simulink library "Clock_Lib"  (R2016a)
settings: Solver=ode45  StartTime=0.0  StopTime=10.0  RelTol=1e-3
libraries: simulink_extras x28
settings Model: Creator=Jozko Mrkvicka  LastModifiedBy=Jozko Mrkvicka
settings DataIOCC: LimitDataPoints=on
settings DebuggingCC: AllowSymbolicDim=off

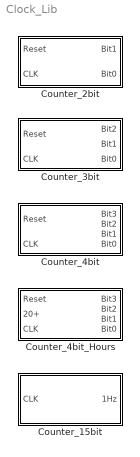
== system Clock_Lib ==
  Counter_15bit : Subsystem
  Counter_2bit : Subsystem
  Counter_3bit : Subsystem
  Counter_4bit : Subsystem
  Counter_4bit_Hours : Subsystem

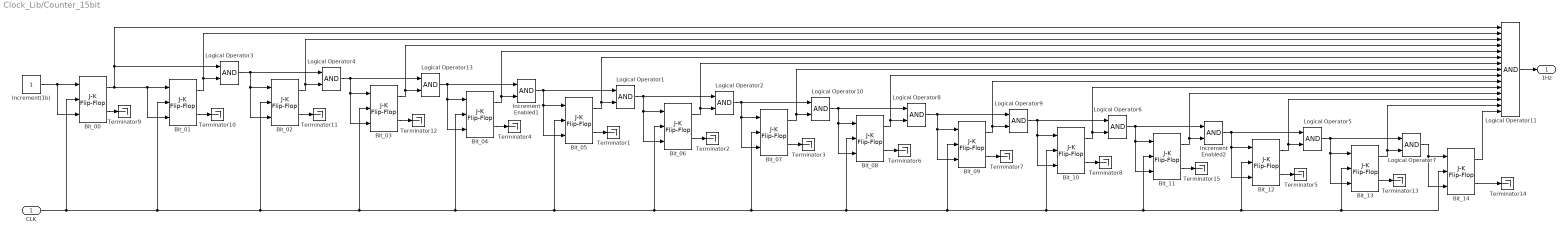
== system Clock_Lib/Counter_15bit ==
  CLK : Inport
  Bit_00 : simulink_extras/Flip Flops/J-K Flip-Flop  initial_condition=0
  Bit_01 : simulink_extras/Flip Flops/J-K Flip-Flop  initial_condition=0
  Bit_02 : simulink_extras/Flip Flops/J-K Flip-Flop  initial_condition=0
  Bit_03 : simulink_extras/Flip Flops/J-K Flip-Flop  initial_condition=0
  Bit_04 : simulink_extras/Flip Flops/J-K Flip-Flop  initial_condition=0
  Bit_05 : simulink_extras/Flip Flops/J-K Flip-Flop  initial_condition=0
  Bit_06 : simulink_extras/Flip Flops/J-K Flip-Flop  initial_condition=0
  Bit_07 : simulink_extras/Flip Flops/J-K Flip-Flop  initial_condition=0
  Bit_08 : simulink_extras/Flip Flops/J-K Flip-Flop  initial_condition=0
  Bit_09 : simulink_extras/Flip Flops/J-K Flip-Flop  initial_condition=0
  Bit_{10..14} (5 alike) : simulink_extras/Flip Flops/J-K Flip-Flop  initial_condition=0
  Increment Enabled1 : Logic  IconShape=distinctive  AllPortsSameDT=off  OutDataTypeStr=boolean
  Increment Enabled2 : Logic  IconShape=distinctive  AllPortsSameDT=off  OutDataTypeStr=boolean
  Increment(1b) : Constant  OutDataTypeStr=boolean
  Logical Operator{1..10,13} (11 alike) : Logic  IconShape=distinctive  AllPortsSameDT=off  OutDataTypeStr=boolean
  Logical Operator11 : Logic  Inputs=15  IconShape=distinctive  AllPortsSameDT=off  OutDataTypeStr=boolean
  Terminator{1..15} (15 alike) : Terminator
  1Hz : Outport
  wires:
  Bit_00/2 -> Terminator9/1
  Increment(1b)/1 -> Bit_00/3, Bit_00/1
  Bit_02/2 -> Terminator11/1
  Bit_03/2 -> Terminator12/1
  Bit_01/2 -> Terminator10/1
  Logical Operator2/1 -> Logical Operator10/1, Bit_07/1, Bit_07/3
  Bit_07/1 -> Logical Operator11/8, Logical Operator10/2
  Bit_06/2 -> Terminator2/1
  Bit_05/2 -> Terminator1/1
  Increment Enabled1/1 -> Bit_05/3, Bit_05/1, Logical Operator1/1
  Bit_07/2 -> Terminator3/1
  Logical Operator13/1 -> Increment Enabled1/1, Bit_04/3, Bit_04/1
  Logical Operator1/1 -> Logical Operator2/1, Bit_06/1, Bit_06/3
  Logical Operator4/1 -> Logical Operator13/1, Bit_03/3, Bit_03/1
  Bit_04/2 -> Terminator4/1
  Logical Operator3/1 -> Logical Operator4/1, Bit_02/3, Bit_02/1
  Bit_09/1 -> Logical Operator11/10, Logical Operator9/2
  Logical Operator10/1 -> Bit_08/1, Bit_08/3, Logical Operator8/1
  Bit_10/1 -> Logical Operator11/11, Logical Operator6/2
  Bit_09/2 -> Terminator7/1
  Bit_10/2 -> Terminator8/1
  Bit_08/2 -> Terminator6/1
  Bit_08/1 -> Logical Operator11/9, Logical Operator8/2
  Bit_13/1 -> Logical Operator11/14, Logical Operator7/2
  Bit_11/1 -> Logical Operator11/12, Increment Enabled2/2
  Bit_12/1 -> Logical Operator11/13, Logical Operator5/2
  Logical Operator7/1 -> Bit_14/1, Bit_14/3
  CLK/1 -> Bit_00/2, Bit_01/2, Bit_02/2, Bit_03/2, Bit_04/2, Bit_05/2, Bit_06/2, Bit_07/2, Bit_08/2, Bit_09/2, Bit_10/2, Bit_11/2, Bit_12/2, Bit_13/2, Bit_14/2
  Bit_14/1 -> Logical Operator11/15
  Bit_13/2 -> Terminator13/1
  Bit_12/2 -> Terminator5/1
  Increment Enabled2/1 -> Bit_12/3, Bit_12/1, Logical Operator5/1
  Bit_14/2 -> Terminator14/1
  Logical Operator6/1 -> Increment Enabled2/1, Bit_11/3, Bit_11/1
  Logical Operator5/1 -> Logical Operator7/1, Bit_13/1, Bit_13/3
  Logical Operator9/1 -> Logical Operator6/1, Bit_10/3, Bit_10/1
  Bit_11/2 -> Terminator15/1
  Logical Operator8/1 -> Logical Operator9/1, Bit_09/3, Bit_09/1
  Bit_06/1 -> Logical Operator11/7, Logical Operator2/2
  Bit_05/1 -> Logical Operator11/6, Logical Operator1/2
  Bit_04/1 -> Logical Operator11/5, Increment Enabled1/2
  Bit_03/1 -> Logical Operator11/4, Logical Operator13/2
  Bit_02/1 -> Logical Operator11/3, Logical Operator4/2
  Bit_01/1 -> Logical Operator11/2, Logical Operator3/2
  Bit_00/1 -> Bit_01/1, Bit_01/3, Logical Operator11/1, Logical Operator3/1
  Logical Operator11/1 -> 1Hz/1

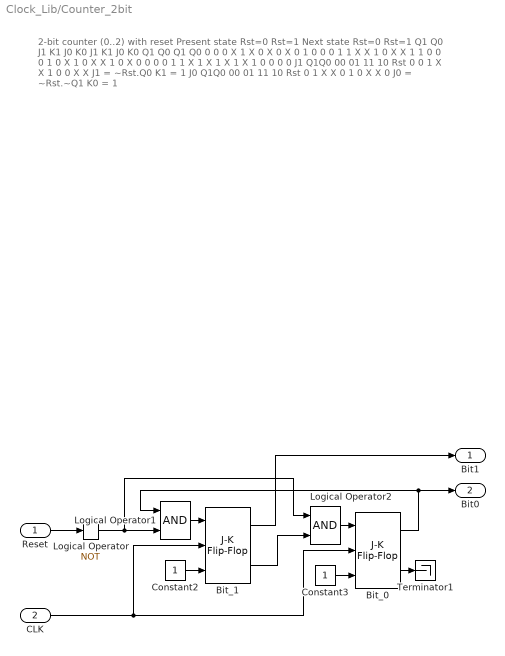
== system Clock_Lib/Counter_2bit ==
  note: 2-bit counter (0..2) with reset
      |
      | Present
      | state
      | Rst=0
      | Rst=1
      | Next state
      |
      | Rst=0
      | Rst=1
      |
      | Q1
      | Q0
      | J1
      | K1
      | J0
      | K0
      | J1
      | K1
      | J0
      | K0
      | Q1
      | Q0
      | Q1
      | Q0
      |
      | 0
      | 0
      | 0
      | X
      | 1
      | X
      | 0
      | X
      | 0
      | X
      | 0
      | 1
      | 0
      | 0
      |
      | 0
      | 1
      | 1
      | X
      | X
      | 1
      | 0
      | X
      | X
      | 1
      | 1
      | 0
      | 0
      | 0
      |
      | 1
      | 0
      | X
      | 1
      | 0
      | X
      | X
      | 1
      | 0
      | X
      | 0
      | 0
      | 0
      | 0
      |
      | 1
      | 1
      | X
      | 1
      | X
      | 1
      | X
      | 1
      | X
      | 1
      | 0
      | 0
      | 0
      | 0
      |
      | J1
      | Q1Q0
      |
      | 00
      | 01
      | 11
      | 10
      |
      | Rst
      | 0
      | 0
      | 1
      | X
      | X
      |
      | 1
      | 0
      | 0
      | X
      | X
      |
      | J1 = ~Rst.Q0
      | K1 = 1
      | J0
      | Q1Q0
      |
      | 00
      | 01
      | 11
      | 10
      |
      | Rst
      | 0
      | 1
      | X
      | X
      | 0
      |
      | 1
      | 0
      | X
      | X
      | 0
      |
      | J0 = ~Rst.~Q1
      | K0 = 1
  Reset : Inport
  CLK : Inport  Port=2
  Bit_0 : simulink_extras/Flip Flops/J-K Flip-Flop  initial_condition=0
  Bit_1 : simulink_extras/Flip Flops/J-K Flip-Flop  initial_condition=0
  Constant2 : Constant  OutDataTypeStr=boolean
  Constant3 : Constant  OutDataTypeStr=boolean
  Logical Operator : Logic  Operator=NOT  IconShape=distinctive  AllPortsSameDT=off  OutDataTypeStr=boolean
  Logical Operator1 : Logic  IconShape=distinctive  AllPortsSameDT=off  OutDataTypeStr=boolean
  Logical Operator2 : Logic  IconShape=distinctive  AllPortsSameDT=off  OutDataTypeStr=boolean
  Terminator1 : Terminator
  Bit1 : Outport
  Bit0 : Outport  Port=2
  wires:
  Constant2/1 -> Bit_1/3
  Constant3/1 -> Bit_0/3
  Bit_0/1 -> Logical Operator1/1, Bit0/1
  Bit_1/2 -> Logical Operator2/2
  CLK/1 -> Bit_0/2, Bit_1/2
  Bit_1/1 -> Bit1/1
  Bit_0/2 -> Terminator1/1
  Logical Operator1/1 -> Bit_1/1
  Reset/1 -> Logical Operator/1
  Logical Operator/1 -> Logical Operator1/2, Logical Operator2/1
  Logical Operator2/1 -> Bit_0/1

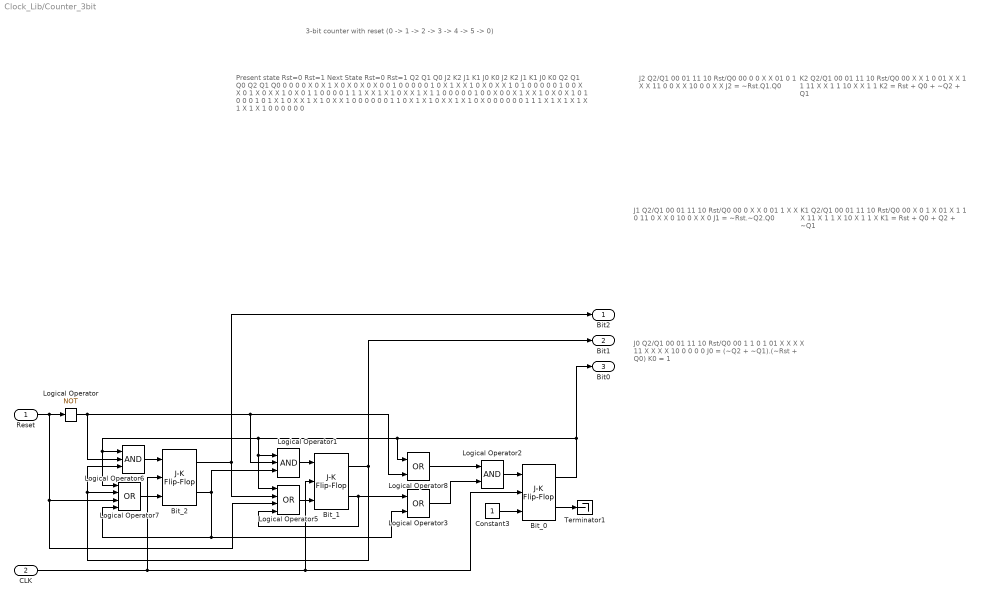
== system Clock_Lib/Counter_3bit ==
  note: J1
      | Q2/Q1
      |
      | 00
      | 01
      | 11
      | 10
      |
      | Rst/Q0
      | 00
      | 0
      | X
      | X
      | 0
      |
      | 01
      | 1
      | X
      | X
      | 0
      |
      | 11
      | 0
      | X
      | X
      | 0
      |
      | 10
      | 0
      | X
      | X
      | 0
      |
      | J1 = ~Rst.~Q2.Q0
  note: J2
      | Q2/Q1
      |
      | 00
      | 01
      | 11
      | 10
      |
      | Rst/Q0
      | 00
      | 0
      | 0
      | X
      | X
      |
      | 01
      | 0
      | 1
      | X
      | X
      |
      | 11
      | 0
      | 0
      | X
      | X
      |
      | 10
      | 0
      | 0
      | X
      | X
      |
      | J2 = ~Rst.Q1.Q0
  note: Present state
      | Rst=0
      | Rst=1
      | Next State
      |
      | Rst=0
      | Rst=1
      |
      | Q2
      | Q1
      | Q0
      | J2
      | K2
      | J1
      | K1
      | J0
      | K0
      | J2
      | K2
      | J1
      | K1
      | J0
      | K0
      | Q2
      | Q1
      | Q0
      | Q2
      | Q1
      | Q0
      |
      | 0
      | 0
      | 0
      | 0
      | X
      | 0
      | X
      | 1
      | X
      | 0
      | X
      | 0
      | X
      | 0
      | X
      | 0
      | 0
      | 1
      | 0
      | 0
      | 0
      |
      | 0
      | 0
      | 1
      | 0
      | X
      | 1
      | X
      | X
      | 1
      | 0
      | X
      | 0
      | X
      | X
      | 1
      | 0
      | 1
      | 0
      | 0
      | 0
      | 0
      |
      | 0
      | 1
      | 0
      | 0
      | X
      | X
      | 0
      | 1
      | X
      | 0
      | X
      | X
      | 1
      | 0
      | X
      | 0
      | 1
      | 1
      | 0
      | 0
      | 0
      |
      | 0
      | 1
      | 1
      | 1
      | X
      | X
      | 1
      | X
      | 1
      | 0
      | X
      | X
      | 1
      | X
      | 1
      | 1
      | 0
      | 0
      | 0
      | 0
      | 0
      |
      | 1
      | 0
      | 0
      | X
      | 0
      | 0
      | X
      | 1
      | X
      | X
      | 1
      | 0
      | X
      | 0
      | X
      | 1
      | 0
      | 1
      | 0
      | 0
      | 0
      |
      | 1
      | 0
      | 1
      | X
      | 1
      | 0
      | X
      | X
      | 1
      | X
      | 1
      | 0
      | X
      | X
      | 1
      | 0
      | 0
      | 0
      | 0
      | 0
      | 0
      |
      | 1
      | 1
      | 0
      | X
      | 1
      | X
      | 1
      | 0
      | X
      | X
      | 1
      | X
      | 1
      | 0
      | X
      | 0
      | 0
      | 0
      | 0
      | 0
      | 0
      |
      | 1
      | 1
      | 1
      | X
      | 1
      | X
      | 1
      | X
      | 1
      | X
      | 1
      | X
      | 1
      | X
      | 1
      | 0
      | 0
      | 0
      | 0
      | 0
      | 0
  note: 3-bit counter with reset
      | (0 -> 1 -> 2 -> 3 -> 4 -> 5 -> 0)
  note: K2
      | Q2/Q1
      |
      | 00
      | 01
      | 11
      | 10
      |
      | Rst/Q0
      | 00
      | X
      | X
      | 1
      | 0
      |
      | 01
      | X
      | X
      | 1
      | 1
      |
      | 11
      | X
      | X
      | 1
      | 1
      |
      | 10
      | X
      | X
      | 1
      | 1
      |
      | K2 = Rst + Q0 + ~Q2 + Q1
  note: K1
      | Q2/Q1
      |
      | 00
      | 01
      | 11
      | 10
      |
      | Rst/Q0
      | 00
      | X
      | 0
      | 1
      | X
      |
      | 01
      | X
      | 1
      | 1
      | X
      |
      | 11
      | X
      | 1
      | 1
      | X
      |
      | 10
      | X
      | 1
      | 1
      | X
      |
      | K1 = Rst + Q0 + Q2 + ~Q1
  note: J0
      | Q2/Q1
      |
      | 00
      | 01
      | 11
      | 10
      |
      | Rst/Q0
      | 00
      | 1
      | 1
      | 0
      | 1
      |
      | 01
      | X
      | X
      | X
      | X
      |
      | 11
      | X
      | X
      | X
      | X
      |
      | 10
      | 0
      | 0
      | 0
      | 0
      |
      | J0 = (~Q2 + ~Q1).(~Rst + Q0)
      | K0 = 1
  Reset : Inport
  CLK : Inport  Port=2
  Bit_0 : simulink_extras/Flip Flops/J-K Flip-Flop  initial_condition=0
  Bit_1 : simulink_extras/Flip Flops/J-K Flip-Flop  initial_condition=0
  Bit_2 : simulink_extras/Flip Flops/J-K Flip-Flop  initial_condition=0
  Constant3 : Constant  OutDataTypeStr=boolean
  Logical Operator : Logic  Operator=NOT  IconShape=distinctive  AllPortsSameDT=off  OutDataTypeStr=boolean
  Logical Operator1 : Logic  Inputs=3  IconShape=distinctive  AllPortsSameDT=off  OutDataTypeStr=boolean
  Logical Operator2 : Logic  IconShape=distinctive  AllPortsSameDT=off  OutDataTypeStr=boolean
  Logical Operator3 : Logic  Operator=OR  IconShape=distinctive  AllPortsSameDT=off  OutDataTypeStr=boolean
  Logical Operator5 : Logic  Operator=OR  Inputs=4  IconShape=distinctive  AllPortsSameDT=off  OutDataTypeStr=boolean
  Logical Operator6 : Logic  Inputs=3  IconShape=distinctive  AllPortsSameDT=off  OutDataTypeStr=boolean
  Logical Operator7 : Logic  Operator=OR  Inputs=4  IconShape=distinctive  AllPortsSameDT=off  OutDataTypeStr=boolean
  Logical Operator8 : Logic  Operator=OR  IconShape=distinctive  AllPortsSameDT=off  OutDataTypeStr=boolean
  Terminator1 : Terminator
  Bit2 : Outport
  Bit1 : Outport  Port=2
  Bit0 : Outport  Port=3
  wires:
  CLK/1 -> Bit_2/2, Bit_1/2, Bit_0/2
  Constant3/1 -> Bit_0/3
  Reset/1 -> Logical Operator/1, Logical Operator5/3, Logical Operator7/3
  Logical Operator/1 -> Logical Operator8/2, Logical Operator1/2, Logical Operator6/2
  Bit_2/1 -> Bit2/1, Logical Operator5/2
  Logical Operator1/1 -> Bit_1/1
  Bit_2/2 -> Logical Operator3/2, Logical Operator7/4, Logical Operator1/3
  Bit_0/1 -> Logical Operator8/1, Logical Operator6/1, Logical Operator7/1, Logical Operator1/1, Logical Operator5/1, Bit0/1
  Logical Operator5/1 -> Bit_1/3
  Bit_1/2 -> Logical Operator3/1, Logical Operator5/4
  Logical Operator6/1 -> Bit_2/1
  Logical Operator7/1 -> Bit_2/3
  Bit_1/1 -> Bit1/1, Logical Operator7/2, Logical Operator6/3
  Logical Operator8/1 -> Logical Operator2/1
  Logical Operator3/1 -> Logical Operator2/2
  Logical Operator2/1 -> Bit_0/1
  Bit_0/2 -> Terminator1/1

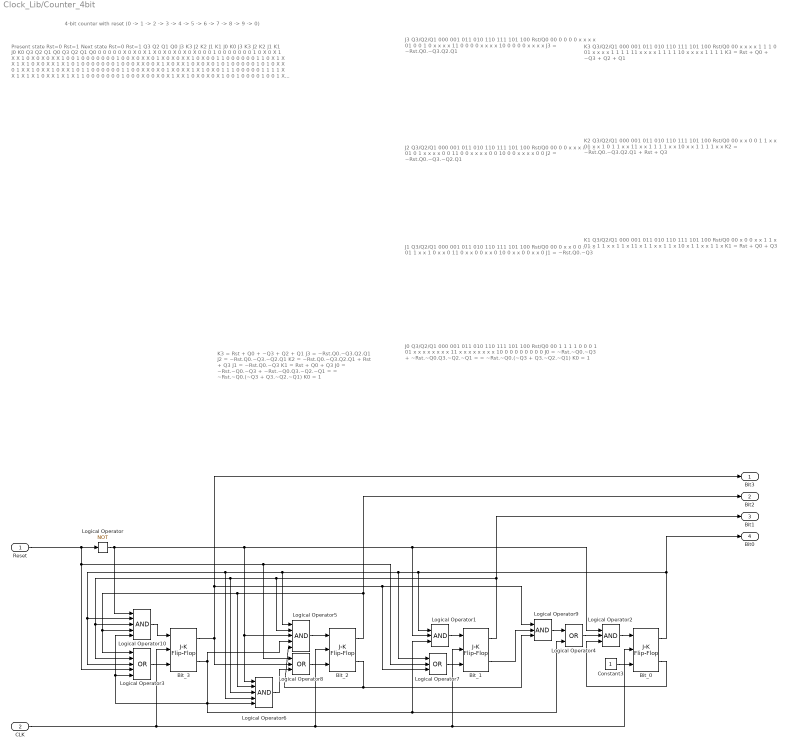
== system Clock_Lib/Counter_4bit ==
  note: K3 = Rst + Q0 + ~Q3 + Q2 + Q1
      | J3 = ~Rst.Q0.~Q3.Q2.Q1
      |
      | J2 = ~Rst.Q0.~Q3.~Q2.Q1
      | K2 = ~Rst.Q0.~Q3.Q2.Q1 + Rst + Q3
      |
      | J1 = ~Rst.Q0.~Q3
      | K1 = Rst + Q0 + Q3
      |
      | J0 = ~Rst.~Q0.~Q3 + ~Rst.~Q0.Q3.~Q2.~Q1 =
      | = ~Rst.~Q0.(~Q3 + Q3.~Q2.~Q1)
      | K0 = 1
  note: Present state
      | Rst=0
      | Rst=1
      | Next state
      |
      | Rst=0
      | Rst=1
      |
      | Q3
      | Q2
      | Q1
      | Q0
      | J3
      | K3
      | J2
      | K2
      | J1
      | K1
      | J0
      | K0
      | J3
      | K3
      | J2
      | K2
      | J1
      | K1
      | J0
      | K0
      | Q3
      | Q2
      | Q1
      | Q0
      | Q3
      | Q2
      | Q1
      | Q0
      |
      | 0
      | 0
      | 0
      | 0
      | 0
      | X
      | 0
      | X
      | 0
      | X
      | 1
      | X
      | 0
      | X
      | 0
      | X
      | 0
      | X
      | 0
      | X
      | 0
      | 0
      | 0
      | 1
      | 0
      | 0
      | 0
      | 0
      |
      | 0
      | 0
      | 0
      | 1
      | 0
      | X
      | 0
      | X
      | 1
      | X
      | X
      | 1
      | 0
      | X
      | 0
      | X
      | 0
      | X
      | X
      | 1
      | 0
      | 0
      | 1
      | 0
      | 0
      | 0
      | 0
      | 0
      |
      | 0
      | 0
      | 1
      | 0
      | 0
      | X
      | 0
      | X
      | X
      | 0
      | 1
      | X
      | 0
      | X
      | 0
      | X
      | X
      | 1
      | 0
      | X
      | 0
      | 0
      | 1
      | 1
      | 0
      | 0
      | 0
      | 0
      |
      | 0
      | 0
      | 1
      | 1
      | 0
      | X
      | 1
      | X
      | X
      | 1
      | X
      | 1
      | 0
      | X
      | 0
      | X
      | X
      | 1
      | X
      | 1
      | 0
      | 1
      | 0
      | 0
      | 0
      | 0
      | 0
      | 0
      |
      | 0
      | 1
      | 0
      | 0
      | 0
      | X
      | X
      | 0
      | 0
      | X
      | 1
      | X
      | 0
      | X
      | X
      | 1
      | 0
      | X
      | 0
      | X
      | 0
      | 1
      | 0
      | 1
      | 0
      | 0
      | 0
      | 0
      |
      | 0
      | 1
      | 0
      | 1
      | 0
      | X
      | X
      | 0
      | 1
      | X
      | X
      | 1
      | 0
      | X
      | X
      | 1
      | 0
      | X
      | X
      | 1
      | 0
      | 1
      | 1
      | 0
      | 0
      | 0
      | 0
      | 0
      |
      | 0
      | 1
      | 1
      | 0
      | 0
      | X
      | X
      | 0
      | X
      | 0
      | 1
      | X
      | 0
      | X
      | X
      | 1
      | X
      | 1
      | 0
      | X
      | 0
      | 1
      | 1
      | 1
      | 0
      | 0
      | 0
      | 0
      |
      | 0
      | 1
      | 1
      | 1
      | 1
      | X
      | X
      | 1
      | X
      | 1
      | X
      | 1
      | 0
      | X
      | X
      | 1
      | X
      | 1
      | X
      | 1
      | 1
      | 0
      | 0
      | 0
      | 0
      | 0
      | 0
      | 0
      |
      | 1
      | 0
      | 0
      | 0
      | X
      | 0
      | 0
      | X
      | 0
      | X
      | 1
      | X
      | X
      | 1
      | 0
      | X
      | 0
      | X
      | 0
      | X
      | 1
      | 0
      | 0
      | 1
      | 0
      | 0
      | 0
      | 0
      |
      | 1
      | 0
      | 0
      | 1
      | X
      | 1
      | 0
      | X
      | 0
      | X
      | X
      | 1
      | X
      | 1
      | 0
      | X
      | 0
      | X
      | X
      | 1
      | 0
      | 0
      | 0
      | 0
      | 0
      | 0
      | 0
      | 0
      |
      | 1
      | 0
      | 1
      | 0
      | X
      | 1
      | 0
      | X
      | X
      | 1
      | 0
      | X
      | X
      | 1
      | 0
      | X
      | X
      | 1
      | 0
      | X
      | 0
      | 0
      | 0
      | 0
      | 0
      | 0
      | 0
      | 0
      |
      | 1
      | 0
      | 1
      | 1
      | X
      | 1
      | 0
      | X
      | X
      | 1
      | X
      | 1
      | X
      | 1
      | 0
      | X
      | X
      | 1
      | X
      | 1
      | 0
      | 0
      | 0
      | 0
      | 0
      | 0
      | 0
      | 0
      |
      | 1
      | 1
      | 0
      | 0
      | X
      | 1
      | X
      | 1
      | 0
      | X
      | 0
      | X
      | X
      | 1
      | X
      | 1
      | 0
      | X
      | 0
      | X
      | 0
      | 0
      | 0
      | 0
      | 0
      | 0
      | 0
      | 0
      |
      | 1
      | 1
      | 0
      | 1
      | X
      | 1
      | X
      | 1
      | 0
      | X
      | X
      | 1
      | X
      | 1
      | X
      | 1
      | 0
      | X
      | X
      | 1
      | 0
      | 0
      | 0
      | 0
      | 0
      | 0
      | 0
      | 0
      |
      | 1
      | 1
      | 1
      | 0
      | X
      | 1
      | X
      | 1
      | X
      | 1
      | 0
      | X
      | X
      | 1
      | X
      | 1
      | X
      | 1
      | 0
      | X
      | 0
      | 0
      | 0
      | 0
      | 0
      | 0
      | 0
      | 0
      |
      | 1
      | 1
      | 1
      | 1
      | X
      | 1
      | X
      | 1
      | X
      | 1
      | X
      | 1
      | X
      | 1
      | X
      | 1
      | X
      | 1
      | X
      | 1
      | 0
      | 0
      | 0
      | 0
      | 0
      | 0
      | 0
      | 0
  note: 4-bit counter with reset
      | (0 -> 1 -> 2 -> 3 -> 4 -> 5 -> 6 -> 7 -> 8 -> 9 -> 0)
  note: K3
      | Q3/Q2/Q1
      |
      | 000
      | 001
      | 011
      | 010
      | 110
      | 111
      | 101
      | 100
      |
      | Rst/Q0
      | 00
      | x
      | x
      | x
      | x
      | 1
      | 1
      | 1
      | 0
      |
      | 01
      | x
      | x
      | x
      | x
      | 1
      | 1
      | 1
      | 1
      |
      | 11
      | x
      | x
      | x
      | x
      | 1
      | 1
      | 1
      | 1
      |
      | 10
      | x
      | x
      | x
      | x
      | 1
      | 1
      | 1
      | 1
      |
      | K3 = Rst + Q0 + ~Q3 + Q2 + Q1
  note: J2
      | Q3/Q2/Q1
      |
      | 000
      | 001
      | 011
      | 010
      | 110
      | 111
      | 101
      | 100
      |
      | Rst/Q0
      | 00
      | 0
      | 0
      | x
      | x
      | x
      | x
      | 0
      | 0
      |
      | 01
      | 0
      | 1
      | x
      | x
      | x
      | x
      | 0
      | 0
      |
      | 11
      | 0
      | 0
      | x
      | x
      | x
      | x
      | 0
      | 0
      |
      | 10
      | 0
      | 0
      | x
      | x
      | x
      | x
      | 0
      | 0
      |
      | J2 = ~Rst.Q0.~Q3.~Q2.Q1
  note: K2
      | Q3/Q2/Q1
      |
      | 000
      | 001
      | 011
      | 010
      | 110
      | 111
      | 101
      | 100
      |
      | Rst/Q0
      | 00
      | x
      | x
      | 0
      | 0
      | 1
      | 1
      | x
      | x
      |
      | 01
      | x
      | x
      | 1
      | 0
      | 1
      | 1
      | x
      | x
      |
      | 11
      | x
      | x
      | 1
      | 1
      | 1
      | 1
      | x
      | x
      |
      | 10
      | x
      | x
      | 1
      | 1
      | 1
      | 1
      | x
      | x
      |
      | K2 = ~Rst.Q0.~Q3.Q2.Q1 + Rst + Q3
  note: J1
      | Q3/Q2/Q1
      |
      | 000
      | 001
      | 011
      | 010
      | 110
      | 111
      | 101
      | 100
      |
      | Rst/Q0
      | 00
      | 0
      | x
      | x
      | 0
      | 0
      | x
      | x
      | 0
      |
      | 01
      | 1
      | x
      | x
      | 1
      | 0
      | x
      | x
      | 0
      |
      | 11
      | 0
      | x
      | x
      | 0
      | 0
      | x
      | x
      | 0
      |
      | 10
      | 0
      | x
      | x
      | 0
      | 0
      | x
      | x
      | 0
      |
      | J1 = ~Rst.Q0.~Q3
  note: K1
      | Q3/Q2/Q1
      |
      | 000
      | 001
      | 011
      | 010
      | 110
      | 111
      | 101
      | 100
      |
      | Rst/Q0
      | 00
      | x
      | 0
      | 0
      | x
      | x
      | 1
      | 1
      | x
      |
      | 01
      | x
      | 1
      | 1
      | x
      | x
      | 1
      | 1
      | x
      |
      | 11
      | x
      | 1
      | 1
      | x
      | x
      | 1
      | 1
      | x
      |
      | 10
      | x
      | 1
      | 1
      | x
      | x
      | 1
      | 1
      | x
      |
      | K1 = Rst + Q0 + Q3
  note: J0
      | Q3/Q2/Q1
      |
      | 000
      | 001
      | 011
      | 010
      | 110
      | 111
      | 101
      | 100
      |
      | Rst/Q0
      | 00
      | 1
      | 1
      | 1
      | 1
      | 0
      | 0
      | 0
      | 1
      |
      | 01
      | x
      | x
      | x
      | x
      | x
      | x
      | x
      | x
      |
      | 11
      | x
      | x
      | x
      | x
      | x
      | x
      | x
      | x
      |
      | 10
      | 0
      | 0
      | 0
      | 0
      | 0
      | 0
      | 0
      | 0
      |
      | J0 = ~Rst.~Q0.~Q3 + ~Rst.~Q0.Q3.~Q2.~Q1 =
      | = ~Rst.~Q0.(~Q3 + Q3.~Q2.~Q1)
      | K0 = 1
  note: J3
      | Q3/Q2/Q1
      |
      | 000
      | 001
      | 011
      | 010
      | 110
      | 111
      | 101
      | 100
      |
      | Rst/Q0
      | 00
      | 0
      | 0
      | 0
      | 0
      | x
      | x
      | x
      | x
      |
      | 01
      | 0
      | 0
      | 1
      | 0
      | x
      | x
      | x
      | x
      |
      | 11
      | 0
      | 0
      | 0
      | 0
      | x
      | x
      | x
      | x
      |
      | 10
      | 0
      | 0
      | 0
      | 0
      | x
      | x
      | x
      | x
      |
      | J3 = ~Rst.Q0.~Q3.Q2.Q1
  Reset : Inport
  CLK : Inport  Port=2
  Bit_{0..3} (4 alike) : simulink_extras/Flip Flops/J-K Flip-Flop  initial_condition=0
  Constant3 : Constant  OutDataTypeStr=boolean
  Logical Operator : Logic  Operator=NOT  IconShape=distinctive  AllPortsSameDT=off  OutDataTypeStr=boolean
  Logical Operator1 : Logic  Inputs=3  IconShape=distinctive  AllPortsSameDT=off  OutDataTypeStr=boolean
  Logical Operator10 : Logic  Inputs=5  IconShape=distinctive  AllPortsSameDT=off  OutDataTypeStr=boolean
  Logical Operator2 : Logic  Inputs=3  IconShape=distinctive  AllPortsSameDT=off  OutDataTypeStr=boolean
  Logical Operator3 : Logic  Operator=OR  Inputs=5  IconShape=distinctive  AllPortsSameDT=off  OutDataTypeStr=boolean
  Logical Operator4 : Logic  Operator=OR  IconShape=distinctive  AllPortsSameDT=off  OutDataTypeStr=boolean
  Logical Operator5 : Logic  Inputs=5  IconShape=distinctive  AllPortsSameDT=off  OutDataTypeStr=boolean
  Logical Operator6 : Logic  Inputs=5  IconShape=distinctive  AllPortsSameDT=off  OutDataTypeStr=boolean
  Logical Operator7 : Logic  Operator=OR  Inputs=3  IconShape=distinctive  AllPortsSameDT=off  OutDataTypeStr=boolean
  Logical Operator8 : Logic  Operator=OR  Inputs=3  IconShape=distinctive  AllPortsSameDT=off  OutDataTypeStr=boolean
  Logical Operator9 : Logic  Inputs=3  IconShape=distinctive  AllPortsSameDT=off  OutDataTypeStr=boolean
  Bit3 : Outport
  Bit2 : Outport  Port=2
  Bit1 : Outport  Port=3
  Bit0 : Outport  Port=4
  wires:
  CLK/1 -> Bit_3/2, Bit_2/2, Bit_1/2, Bit_0/2
  Constant3/1 -> Bit_0/3
  Logical Operator10/1 -> Bit_3/1
  Logical Operator3/1 -> Bit_3/3
  Bit_3/2 -> Logical Operator5/4, Logical Operator1/3, Logical Operator4/2, Logical Operator6/5, Logical Operator3/5, Logical Operator10/5
  Bit_2/1 -> Bit2/1, Logical Operator6/2, Logical Operator3/1, Logical Operator10/4
  Bit_0/1 -> Bit0/1, Logical Operator1/1, Logical Operator7/1, Logical Operator5/1, Logical Operator6/4, Logical Operator10/2, Logical Operator3/3
  Logical Operator/1 -> Logical Operator10/1, Logical Operator2/1, Logical Operator1/2, Logical Operator5/3, Logical Operator6/1
  Logical Operator5/1 -> Bit_2/1
  Bit_2/2 -> Logical Operator5/5, Logical Operator9/3
  Logical Operator8/1 -> Bit_2/3
  Bit_3/1 -> Bit3/1, Logical Operator7/3, Logical Operator9/1, Logical Operator8/2
  Logical Operator6/1 -> Logical Operator8/3
  Bit_1/1 -> Bit1/1, Logical Operator5/2, Logical Operator10/3, Logical Operator3/2, Logical Operator6/3
  Logical Operator1/1 -> Bit_1/1
  Logical Operator7/1 -> Bit_1/3
  Reset/1 -> Logical Operator/1, Logical Operator7/2, Logical Operator8/1, Logical Operator3/4
  Logical Operator4/1 -> Logical Operator2/2
  Logical Operator2/1 -> Bit_0/1
  Bit_0/2 -> Logical Operator2/3
  Logical Operator9/1 -> Logical Operator4/1
  Bit_1/2 -> Logical Operator9/2

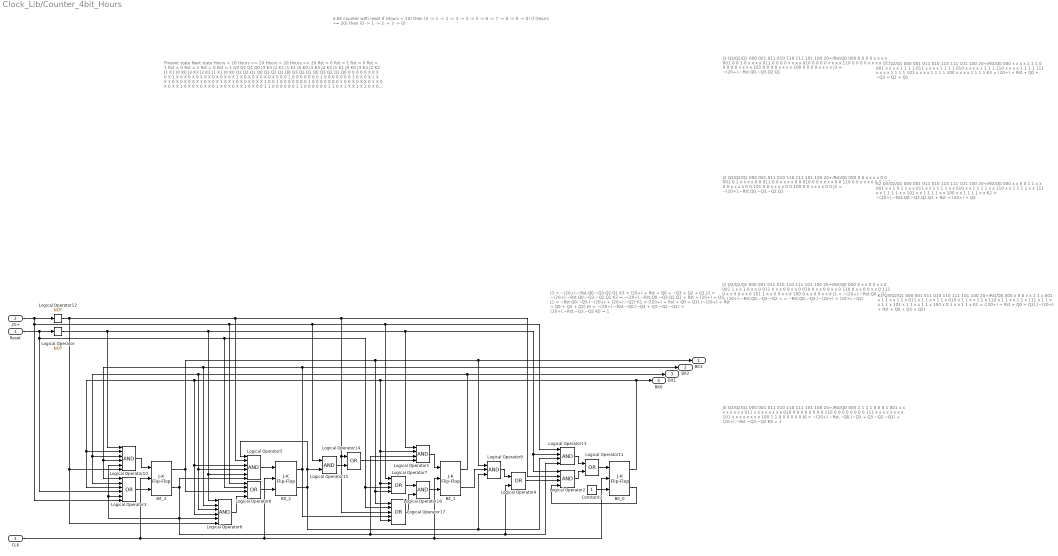
== system Clock_Lib/Counter_4bit_Hours ==
  note: J3 = ~(20+).~Rst.Q0.~Q3.Q2.Q1
      | K3 = (20+) + Rst + Q0 + ~Q3 + Q2 + Q1
      |
      | J2 = ~(20+).~Rst.Q0.~Q3.~Q2.Q1
      | K2 = ~(20+).~Rst.Q0.~Q3.Q2.Q1 + Rst + (20+) + Q3
      |
      | J1 = ~Rst.Q0.~Q3.(~(20+) + (20+).~Q2)
      | K1 = ((20+) + Rst + Q0 + Q3).(~(20+) + Rst + Q0 + Q3 + Q2)
      |
      | J0 = ~(20+).~Rst.~Q0.(~Q3 + Q3.~Q2.~Q1) + (20+).~Rst.~Q3.~Q2
      | K0 = 1
  note: Present state
      |
      | Next state
      |
      | Hours < 20
      | Hours >= 20
      | Hours < 20
      | Hours >= 20
      |
      | Rst = 0
      | Rst = 1
      | Rst = 0
      | Rst = 1
      | Rst = 0
      | Rst = 1
      | Rst = 0
      | Rst = 1
      |
      | Q3
      | Q2
      | Q1
      | Q0
      | J3
      | K3
      | J2
      | K2
      | J1
      | K1
      | J0
      | K0
      | J3
      | K3
      | J2
      | K2
      | J1
      | K1
      | J0
      | K0
      | J3
      | K3
      | J2
      | K2
      | J1
      | K1
      | J0
      | K0
      | J3
      | K3
      | J2
      | K2
      | J1
      | K1
      | J0
      | K0
      | Q3
      | Q2
      | Q1
      | Q0
      | Q3
      | Q2
      | Q1
      | Q0
      | Q3
      | Q2
      | Q1
      | Q0
      | Q3
      | Q2
      | Q1
      | Q0
      |
      | 0
      | 0
      | 0
      | 0
      | 0
      | X
      | 0
      | X
      | 0
      | X
      | 1
      | X
      | 0
      | X
      | 0
      | X
      | 0
      | X
      | 0
      | X
      | 0
      | X
      | 0
      | X
      | 0
      | X
      | 1
      | X
      | 0
      | X
      | 0
      | X
      | 0
      | X
      | 0
      | X
      | 0
      | 0
      | 0
      | 1
      | 0
      | 0
      | 0
      | 0
      | 0
      | 0
      | 0
      | 1
      | 0
      | 0
      | 0
      | 0
      |
      | 0
      | 0
      | 0
      | 1
      | 0
      | X
      | 0
      | X
      | 1
      | X
      | X
      | 1
      | 0
      | X
      | 0
      | X
      | 0
      | X
      | X
      | 1
      | 0
      | X
      | 0
      | X
      | 1
      | X
      | X
      | 1
      | 0
      | X
      | 0
      | X
      | 0
      | X
      | X
      | 1
      | 0
      | 0
      | 1
      | 0
      | 0
      | 0
      | 0
      | 0
      | 0
      | 0
      | 1
      | 0
      | 0
      | 0
      | 0
      | 0
      |
      | 0
      | 0
      | 1
      | 0
      | 0
      | X
      | 0
      | X
      | X
      | 0
      | 1
      | X
      | 0
      | X
      | 0
      | X
      | X
      | 1
      | 0
      | X
      | 0
      | X
      | 0
      | X
      | X
      | 0
      | 1
      | X
      | 0
      | X
      | 0
      | X
      | X
      | 1
      | 0
      | X
      | 0
      | 0
      | 1
      | 1
      | 0
      | 0
      | 0
      | 0
      | 0
      | 0
      | 1
      | 1
      | 0
      | 0
      | 0
      | 0
      |
      | 0
      | 0
      | 1
      | 1
      | 0
      | X
      | 1
      | X
      | X
      | 1
      | X
      | 1
      | 0
      | X
      | 0
      | X
      | X
      | 1
      | X
      | 1
      | 0
      | X
      | 0
      | X
      | X
      | 1
      | X
      | 1
      | 0
      | X
      | 0
      | X
      | X
      | 1
      | X
      | 1
      | 0
      | 1
      | 0
      | 0
      | 0
      | 0
      | 0
      | 0
      | 0
      | 0
      | 0
      | 0
      | 0
      | 0
      | 0
      | 0
      |
      | 0
      | 1
      | 0
      | 0
      | 0
      | X
      | X
      | 0
      | 0
      | X
      | 1
      | X
      | 0
      | X
      | X
      | 1
      | 0
      | X
      | 0
      | X
      | 0
      | X
      | X
      | 1
      | 0
      | X
      | 0
      | X
      | 0
      | X
      | X
      | 1
      | 0
      | X
      | 0
      | X
      | 0
      | 1
      | 0
      | 1
      | 0
      | 0
      | 0
      | 0
      | 0
      | 0
      | 0
      | 0
      | 0
      | 0
      | 0
      | 0
      |
      | 0
      | 1
      | 0
      | 1
      | 0
      | X
      | X
      | 0
      | 1
      | X
      | X
      | 1
      | 0
      | X
      | X
      | 1
      | 0
      | X
      | X
      | 1
      | 0
      | X
      | X
      | 1
      | 0
      | X
      | X
      | 1
      | 0
      | X
      | X
      | 1
      | 0
      | X
      | X
      | 1
      | 0
      | 1
      | 1
      | 0
      | 0
      | 0
      | 0
      | 0
      | 0
      | 0
      | 0
      | 0
      | 0
      | 0
      | 0
      | 0
      |
      | 0
      | 1
      | 1
      | 0
      | 0
      | X
      | X
      | 0
      | X
      | 0
      | 1
      | X
      | 0
      | X
      | X
      | 1
      | X
      | 1
      | 0
      | X
      | 0
      | X
      | X
      | 1
      | X
      | 1
      | 0
      | X
      | 0
      | X
      | X
      | 1
      | X
      | 1
      | 0
      | X
      | 0
      | 1
      | 1
      | 1
      | 0
      | 0
      | 0
      | 0
      | 0
      | 0
      | 0
      | 0
      | 0
      | 0
      | 0
      | 0
      |
      | 0
      | 1
      | 1
      | 1
      | 1
      | X
      | X
      | 1
      | X
      | 1
      | X
      | 1
      | 0
      | X
      | X
      | 1
      | X
      | 1
      | X
      | 1
      | 0
      | X
      | X
      | 1
      | X
      | 1
      | X
      | 1
      | 0
      | X
      | X
      | 1
      | X
      | 1
      | X
      | 1
      | 1
      | 0
      | 0
      | 0
      | 0
      | 0
      | 0
      | 0
      | 0
      | 0
      | 0
      | 0
      | 0
      | 0
      | 0
      | 0
      |
      | 1
      | 0
      | 0
      | 0
      | X
      | 0
      | 0
      | X
      | 0
      | X
      | 1
      | X
      | X
      | 1
      | 0
      | X
      | 0
      | X
      | 0
      | X
      | X
      | 1
      | 0
      | X
      | 0
      | X
      | 0
      | X
      | X
      | 1
      | 0
      | X
      | 0
      | X
      | 0
      | X
      | 1
      | 0
      | 0
      | 1
      | 0
      | 0
      | 0
      | 0
      | 0
      | 0
      | 0
      | 0
      | 0
      | 0
      | 0
      | 0
      |
      | 1
      | 0
      | 0
      | 1
      | X
      | 1
      | 0
      | X
      | 0
      | X
      | X
      | 1
      | X
      | 1
      | 0
      | X
      | 0
      | X
      | X
      | 1
      | X
      | 1
      | 0
      | X
      | 0
      | X
      | X
      | 1
      | X
      | 1
      | 0
      | X
      | 0
      | X
      | X
      | 1
      | 0
      | 0
      | 0
      | 0
      | 0
      | 0
      | 0
      | 0
      | 0
      | 0
      | 0
      | 0
      | 0
      | 0
      | 0
      | 0
      |
      | 1
      | 0
      | 1
      | 0
      | X
      | 1
      | 0
      | X
      | X
      | 1
      | 0
      | X
      | X
      | 1
      | 0
      | X
      | X
      | 1
      | 0
      | X
      | X
      | 1
      | 0
      | X
      | X
      | 1
      | 0
      | X
      | X
      | 1
      | 0
      | X
      | X
      | 1
      | 0
      | X
      | 0
      | 0
      | 0
      | 0
      | 0
      | 0
      | 0
      | 0
      | 0
      | 0
      | 0
      | 0
      | 0
      | 0
      | 0
      | 0
      |
      | 1
      | 0
      | 1
      | 1
      | X
      | 1
      | 0
      | X
      | X
      | 1
      | X
      | 1
      | X
      | 1
      | 0
      | X
      | X
      | 1
      | X
      | 1
      | X
      | 1
      | 0
      | X
      | X
      | 1
      | X
      | 1
      | X
      | 1
      | 0
      | X
      | X
      | 1
      | X
      | 1
      | 0
      | 0
      | 0
      | 0
      | 0
      | 0
      | 0
      | 0
      | 0
      | 0
      | 0
      | 0
      | 0
      | 0
      | 0
      | 0
      |
      | 1
      | 1
      | 0
      | 0
      | X
      | 1
      | X
      | 1
      | 0
      | X
      | 0
      | X
      | X
      | 1
      | X
      | 1
      | 0
      | X
      | 0
      | X
      | X
      | 1
      | X
      | 1
      | 0
      | X
      | 0
      | X
      | X
      | 1
      | X
      | 1
      | 0
      | X
      | 0
      | X
      | 0
      | 0
      | 0
      | 0
      | 0
      | 0
      | 0
      | 0
      | 0
      | 0
      | 0
      | 0
      | 0
      | 0
      | 0
      | 0
      |
      | 1
      | 1
      | 0
      | 1
      | X
      | 1
      | X
      | 1
      | 0
      | X
      | X
      | 1
      | X
      | 1
      | X
      | 1
      | 0
      | X
      | X
      | 1
      | X
      | 1
      | X
      | 1
      | 0
      | X
      | X
      | 1
      | X
      | 1
      | X
      | 1
      | 0
      | X
      | X
      | 1
      | 0
      | 0
      | 0
      | 0
      | 0
      | 0
      | 0
      | 0
      | 0
      | 0
      | 0
      | 0
      | 0
      | 0
      | 0
      | 0
      |
      | 1
      | 1
      | 1
      | 0
      | X
      | 1
      | X
      | 1
      | X
      | 1
      | 0
      | X
      | X
      | 1
      | X
      | 1
      | X
      | 1
      | 0
      | X
      | X
      | 1
      | X
      | 1
      | X
      | 1
      | 0
      | X
      | X
      | 1
      | X
      | 1
      | X
      | 1
      | 0
      | X
      | 0
      | 0
      | 0
      | 0
      | 0
      | 0
      | 0
      | 0
      | 0
      | 0
      | 0
      | 0
      | 0
      | 0
      | 0
      | 0
      |
      | 1
      | 1
      | 1
      | 1
      | X
      | 1
      | X
      | 1
      | X
      | 1
      | X
      | 1
      | X
      | 1
      | X
      | 1
      | X
      | 1
      | X
      | 1
      | X
      | 1
      | X
      | 1
      | X
      | 1
      | X
      | 1
      | X
      | 1
      | X
      | 1
      | X
      | 1
      | X
      | 1
      | 0
      | 0
      | 0
      | 0
      | 0
      | 0
      | 0
      | 0
      | 0
      | 0
      | 0
      | 0
      | 0
      | 0
      | 0
      | 0
  note: 4-bit counter with reset
      | If (Hours < 20) then
      | (0 -> 1 -> 2 -> 3 -> 4 -> 5 -> 6 -> 7 -> 8 -> 9 -> 0)
      |
      | If (Hours >= 20) then
      | (0 -> 1 -> 2 -> 3 -> 0)
  note: K3
      | Q3/Q2/Q1
      |
      | 000
      | 001
      | 011
      | 010
      | 110
      | 111
      | 101
      | 100
      |
      | 20+/Rst/Q0
      | 000
      | x
      | x
      | x
      | x
      | 1
      | 1
      | 1
      | 0
      |
      | 001
      | x
      | x
      | x
      | x
      | 1
      | 1
      | 1
      | 1
      |
      | 011
      | x
      | x
      | x
      | x
      | 1
      | 1
      | 1
      | 1
      |
      | 010
      | x
      | x
      | x
      | x
      | 1
      | 1
      | 1
      | 1
      |
      | 110
      | x
      | x
      | x
      | x
      | 1
      | 1
      | 1
      | 1
      |
      | 111
      | x
      | x
      | x
      | x
      | 1
      | 1
      | 1
      | 1
      |
      | 101
      | x
      | x
      | x
      | x
      | 1
      | 1
      | 1
      | 1
      |
      | 100
      | x
      | x
      | x
      | x
      | 1
      | 1
      | 1
      | 1
      |
      | K3 = (20+) + Rst + Q0 + ~Q3 + Q2 + Q1
  note: J2
      | Q3/Q2/Q1
      |
      | 000
      | 001
      | 011
      | 010
      | 110
      | 111
      | 101
      | 100
      |
      | 20+/Rst/Q0
      | 000
      | 0
      | 0
      | x
      | x
      | x
      | x
      | 0
      | 0
      |
      | 001
      | 0
      | 1
      | x
      | x
      | x
      | x
      | 0
      | 0
      |
      | 011
      | 0
      | 0
      | x
      | x
      | x
      | x
      | 0
      | 0
      |
      | 010
      | 0
      | 0
      | x
      | x
      | x
      | x
      | 0
      | 0
      |
      | 110
      | 0
      | 0
      | x
      | x
      | x
      | x
      | 0
      | 0
      |
      | 111
      | 0
      | 0
      | x
      | x
      | x
      | x
      | 0
      | 0
      |
      | 101
      | 0
      | 0
      | x
      | x
      | x
      | x
      | 0
      | 0
      |
      | 100
      | 0
      | 0
      | x
      | x
      | x
      | x
      | 0
      | 0
      |
      | J2 = ~(20+).~Rst.Q0.~Q3.~Q2.Q1
  note: K2
      | Q3/Q2/Q1
      |
      | 000
      | 001
      | 011
      | 010
      | 110
      | 111
      | 101
      | 100
      |
      | 20+/Rst/Q0
      | 000
      | x
      | x
      | 0
      | 0
      | 1
      | 1
      | x
      | x
      |
      | 001
      | x
      | x
      | 1
      | 0
      | 1
      | 1
      | x
      | x
      |
      | 011
      | x
      | x
      | 1
      | 1
      | 1
      | 1
      | x
      | x
      |
      | 010
      | x
      | x
      | 1
      | 1
      | 1
      | 1
      | x
      | x
      |
      | 110
      | x
      | x
      | 1
      | 1
      | 1
      | 1
      | x
      | x
      |
      | 111
      | x
      | x
      | 1
      | 1
      | 1
      | 1
      | x
      | x
      |
      | 101
      | x
      | x
      | 1
      | 1
      | 1
      | 1
      | x
      | x
      |
      | 100
      | x
      | x
      | 1
      | 1
      | 1
      | 1
      | x
      | x
      |
      | K2 = ~(20+).~Rst.Q0.~Q3.Q2.Q1 + Rst + (20+) + Q3
  note: J1
      | Q3/Q2/Q1
      |
      | 000
      | 001
      | 011
      | 010
      | 110
      | 111
      | 101
      | 100
      |
      | 20+/Rst/Q0
      | 000
      | 0
      | x
      | x
      | 0
      | 0
      | x
      | x
      | 0
      |
      | 001
      | 1
      | x
      | x
      | 1
      | 0
      | x
      | x
      | 0
      |
      | 011
      | 0
      | x
      | x
      | 0
      | 0
      | x
      | x
      | 0
      |
      | 010
      | 0
      | x
      | x
      | 0
      | 0
      | x
      | x
      | 0
      |
      | 110
      | 0
      | x
      | x
      | 0
      | 0
      | x
      | x
      | 0
      |
      | 111
      | 0
      | x
      | x
      | 0
      | 0
      | x
      | x
      | 0
      |
      | 101
      | 1
      | x
      | x
      | 0
      | 0
      | x
      | x
      | 0
      |
      | 100
      | 0
      | x
      | x
      | 0
      | 0
      | x
      | x
      | 0
      |
      | J1 = ~(20+).~Rst.Q0.~Q3 + (20+).~Rst.Q0.~Q3.~Q2 =
      | = ~Rst.Q0.~Q3.(~(20+) + (20+).~Q2)
  note: K1
      | Q3/Q2/Q1
      |
      | 000
      | 001
      | 011
      | 010
      | 110
      | 111
      | 101
      | 100
      |
      | 20+/Rst/Q0
      | 000
      | x
      | 0
      | 0
      | x
      | x
      | 1
      | 1
      | x
      |
      | 001
      | x
      | 1
      | 1
      | x
      | x
      | 1
      | 1
      | x
      |
      | 011
      | x
      | 1
      | 1
      | x
      | x
      | 1
      | 1
      | x
      |
      | 010
      | x
      | 1
      | 1
      | x
      | x
      | 1
      | 1
      | x
      |
      | 110
      | x
      | 1
      | 1
      | x
      | x
      | 1
      | 1
      | x
      |
      | 111
      | x
      | 1
      | 1
      | x
      | x
      | 1
      | 1
      | x
      |
      | 101
      | x
      | 1
      | 1
      | x
      | x
      | 1
      | 1
      | x
      |
      | 100
      | x
      | 0
      | 1
      | x
      | x
      | 1
      | 1
      | x
      |
      | K1 = ((20+) + Rst + Q0 + Q3).(~(20+) + Rst + Q0 + Q3 + Q2)
  note: J0
      | Q3/Q2/Q1
      |
      | 000
      | 001
      | 011
      | 010
      | 110
      | 111
      | 101
      | 100
      |
      | 20+/Rst/Q0
      | 000
      | 1
      | 1
      | 1
      | 1
      | 0
      | 0
      | 0
      | 1
      |
      | 001
      | x
      | x
      | x
      | x
      | x
      | x
      | x
      | x
      |
      | 011
      | x
      | x
      | x
      | x
      | x
      | x
      | x
      | x
      |
      | 010
      | 0
      | 0
      | 0
      | 0
      | 0
      | 0
      | 0
      | 0
      |
      | 110
      | 0
      | 0
      | 0
      | 0
      | 0
      | 0
      | 0
      | 0
      |
      | 111
      | x
      | x
      | x
      | x
      | x
      | x
      | x
      | x
      |
      | 101
      | x
      | x
      | x
      | x
      | x
      | x
      | x
      | x
      |
      | 100
      | 1
      | 1
      | 0
      | 0
      | 0
      | 0
      | 0
      | 0
      |
      | J0 = ~(20+).~Rst.~Q0.(~Q3 + Q3.~Q2.~Q1) + (20+).~Rst.~Q3.~Q2
      | K0 = 1
  note: J3
      | Q3/Q2/Q1
      |
      | 000
      | 001
      | 011
      | 010
      | 110
      | 111
      | 101
      | 100
      |
      | 20+/Rst/Q0
      | 000
      | 0
      | 0
      | 0
      | 0
      | x
      | x
      | x
      | x
      |
      | 001
      | 0
      | 0
      | 1
      | 0
      | x
      | x
      | x
      | x
      |
      | 011
      | 0
      | 0
      | 0
      | 0
      | x
      | x
      | x
      | x
      |
      | 010
      | 0
      | 0
      | 0
      | 0
      | x
      | x
      | x
      | x
      |
      | 110
      | 0
      | 0
      | 0
      | 0
      | x
      | x
      | x
      | x
      |
      | 111
      | 0
      | 0
      | 0
      | 0
      | x
      | x
      | x
      | x
      |
      | 101
      | 0
      | 0
      | 0
      | 0
      | x
      | x
      | x
      | x
      |
      | 100
      | 0
      | 0
      | 0
      | 0
      | x
      | x
      | x
      | x
      |
      | J3 = ~(20+).~Rst.Q0.~Q3.Q2.Q1
  Reset : Inport
  20+ : Inport  Port=2
  CLK : Inport  Port=3
  Bit_{0..3} (4 alike) : simulink_extras/Flip Flops/J-K Flip-Flop  initial_condition=0
  Constant3 : Constant  OutDataTypeStr=boolean
  Logical Operator : Logic  Operator=NOT  IconShape=distinctive  AllPortsSameDT=off  OutDataTypeStr=boolean
  Logical Operator1 : Logic  Inputs=4  IconShape=distinctive  AllPortsSameDT=off  OutDataTypeStr=boolean
  Logical Operator10 : Logic  Inputs=6  IconShape=distinctive  AllPortsSameDT=off  OutDataTypeStr=boolean
  Logical Operator11 : Logic  Operator=OR  IconShape=distinctive  AllPortsSameDT=off  OutDataTypeStr=boolean
  Logical Operator12 : Logic  Operator=NOT  IconShape=distinctive  AllPortsSameDT=off  OutDataTypeStr=boolean
  Logical Operator13 : Logic  Inputs=4  IconShape=distinctive  AllPortsSameDT=off  OutDataTypeStr=boolean
  Logical Operator14 : Logic  Operator=OR  IconShape=distinctive  AllPortsSameDT=off  OutDataTypeStr=boolean
  Logical Operator15 : Logic  IconShape=distinctive  AllPortsSameDT=off  OutDataTypeStr=boolean
  Logical Operator16 : Logic  IconShape=distinctive  AllPortsSameDT=off  OutDataTypeStr=boolean
  Logical Operator17 : Logic  Operator=OR  Inputs=5  IconShape=distinctive  AllPortsSameDT=off  OutDataTypeStr=boolean
  Logical Operator2 : Logic  Inputs=4  IconShape=distinctive  AllPortsSameDT=off  OutDataTypeStr=boolean
  Logical Operator3 : Logic  Operator=OR  Inputs=6  IconShape=distinctive  AllPortsSameDT=off  OutDataTypeStr=boolean
  Logical Operator4 : Logic  Operator=OR  IconShape=distinctive  AllPortsSameDT=off  OutDataTypeStr=boolean
  Logical Operator5 : Logic  Inputs=6  IconShape=distinctive  AllPortsSameDT=off  OutDataTypeStr=boolean
  Logical Operator6 : Logic  Inputs=6  IconShape=distinctive  AllPortsSameDT=off  OutDataTypeStr=boolean
  Logical Operator7 : Logic  Operator=OR  Inputs=4  IconShape=distinctive  AllPortsSameDT=off  OutDataTypeStr=boolean
  Logical Operator8 : Logic  Operator=OR  Inputs=4  IconShape=distinctive  AllPortsSameDT=off  OutDataTypeStr=boolean
  Logical Operator9 : Logic  Inputs=3  IconShape=distinctive  AllPortsSameDT=off  OutDataTypeStr=boolean
  Bit3 : Outport
  Bit2 : Outport  Port=2
  Bit1 : Outport  Port=3
  Bit0 : Outport  Port=4
  wires:
  CLK/1 -> Bit_3/2, Bit_2/2, Bit_1/2, Bit_0/2
  Constant3/1 -> Bit_0/3
  Logical Operator10/1 -> Bit_3/1
  Logical Operator3/1 -> Bit_3/3
  Bit_3/2 -> Logical Operator5/6, Logical Operator1/3, Logical Operator4/2, Logical Operator13/4, Logical Operator3/5, Logical Operator10/5, Logical Operator6/5
  Bit_2/1 -> Logical Operator6/2, Logical Operator3/1, Logical Operator10/4, Bit2/1, Logical Operator17/4
  Bit_0/1 -> Logical Operator7/2, Logical Operator17/5, Logical Operator1/2, Logical Operator5/3, Logical Operator6/4, Logical Operator3/3, Logical Operator10/2, Bit0/1
  Logical Operator/1 -> Logical Operator10/1, Logical Operator5/5, Logical Operator6/1, Logical Operator1/1, Logical Operator2/1, Logical Operator13/2
  Logical Operator5/1 -> Bit_2/1
  Bit_2/2 -> Logical Operator5/1, Logical Operator15/2, Logical Operator9/3, Logical Operator13/3
  Logical Operator8/1 -> Bit_2/3
  Bit_3/1 -> Logical Operator8/3, Logical Operator7/4, Logical Operator17/1, Logical Operator9/1, Bit3/1
  Logical Operator6/1 -> Logical Operator8/4
  Bit_1/1 -> Logical Operator5/4, Logical Operator6/3, Logical Operator3/2, Logical Operator10/3, Bit1/1
  Logical Operator1/1 -> Bit_1/1
  Logical Operator7/1 -> Logical Operator16/1
  Reset/1 -> Logical Operator/1, Logical Operator3/4, Logical Operator8/2, Logical Operator17/2, Logical Operator7/3
  Logical Operator4/1 -> Logical Operator2/3
  Logical Operator2/1 -> Logical Operator11/2
  Bit_0/2 -> Logical Operator2/4
  Logical Operator9/1 -> Logical Operator4/1
  Bit_1/2 -> Logical Operator9/2
  Logical Operator11/1 -> Bit_0/1
  20+/1 -> Logical Operator12/1, Logical Operator8/1, Logical Operator15/1, Logical Operator7/1, Logical Operator13/1, Logical Operator3/6
  Logical Operator12/1 -> Logical Operator17/3, Logical Operator14/1, Logical Operator2/2, Logical Operator5/2, Logical Operator6/6, Logical Operator10/6
  Logical Operator13/1 -> Logical Operator11/1
  Logical Operator14/1 -> Logical Operator1/4
  Logical Operator15/1 -> Logical Operator14/2
  Logical Operator16/1 -> Bit_1/3
  Logical Operator17/1 -> Logical Operator16/2
